simulink model "untitled"  (Simulink 8.6)
settings: Solver=FixedStepDiscrete  StartTime=0.0  StopTime=10.0  FixedStep=0.01  RelTol=1e-3
undefined symbols (not defined in the file or in its folder): DiscIntNeverNeededParam
settings Model: Creator=Igor  LastModifiedBy=User
settings DebuggingCC: FcnCallInpInsideContextMsg=EnableAllAsWarning
settings GRTTargetCC: CombineOutputUpdateFcns=on  GRTInterface=off

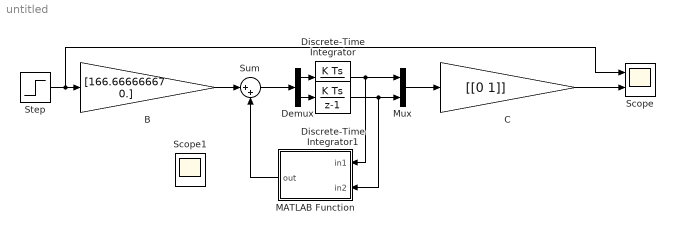
== system untitled ==
  B : Gain  Gain=[166.66666667 0.]  SampleTime=0.01
  C : Gain  Gain=[[0 1]]  SampleTime=0.01
  Demux : Demux  Outputs=2
  Discrete-Time Integrator : DiscreteIntegrator  SampleTime=0.01  ICPrevOutput=DiscIntNeverNeededParam  ICPrevScaledInput=DiscIntNeverNeededParam
  Discrete-Time Integrator1 : DiscreteIntegrator  SampleTime=0.01  ICPrevOutput=DiscIntNeverNeededParam  ICPrevScaledInput=DiscIntNeverNeededParam
  MATLAB Function : MATLAB Function  TreatAsAtomicUnit=on
  Mux : Mux  Inputs=2
  Scope : Scope  NumInputPorts=2
  Scope1 : Scope  NumInputPorts=2
  Step : Step  After=-1  SampleTime=0
  Sum : Sum  Inputs=|++
  wires:
  Step/1 -> B/1, Scope/1
  C/1 -> Scope/2
  Demux/1 -> Discrete-Time Integrator/1
  Demux/2 -> Discrete-Time Integrator1/1
  Discrete-Time Integrator/1 -> MATLAB Function/1(in1), Mux/1
  Discrete-Time Integrator1/1 -> MATLAB Function/2(in2), Mux/2
  B/1 -> Sum/1
  Sum/1 -> Demux/1
  Mux/1 -> C/1
  MATLAB Function/1(out) -> Sum/2

== matlab function MATLAB Function ==
  data: in1 input double; out output double; in2 input double
function out = fcn(in1,in2)

  Abrakadbra10100500 = [-33.33333333 -216.66666667 ; 13. 0.];
  out = [in1 in2]*(Abrakadbra10100500);
